simulink model "least_square_p3_3ordem"  (Simulink 10.3)
settings: Solver=VariableStepAuto  StartTime=0.0  StopTime=10.0  RelTol=1e-3
values from neighbouring files (symbols this model uses):
  Aq = 2    [sim_grad_norm_3ordem.m]
  As = 2    [sim_grad_norm.m]    (also in sim_grad_norm_3ordem.m = 0)
  DC = 1    [sim_grad_norm.m]    (also in sim_grad_norm_3ordem.m)
  kappa = 1e-9    (= 1e-09)    [sim_grad_norm.m]    (also in sim_grad_norm_3ordem.m = 1)
  lambda0 = 1    [sim_grad_norm.m]    (also in sim_grad_norm_3ordem.m)
  lambda1 = 2    [sim_grad_norm.m]    (also in sim_grad_norm_3ordem.m)
  lambda2 = 3    [sim_grad_norm.m]    (also in sim_grad_norm_3ordem.m)
  P0 = eye(6)    [sim_grad_norm.m]    (also in sim_grad_norm_3ordem.m = 1*eye(6))
  st = 0.01    [sim_grad_norm.m]    (also in sim_grad_norm_3ordem.m)
  theta0 = [0;0;0;0;0;0]    [sim_grad_norm.m]    (also in sim_grad_norm_3ordem.m)
  theta_star2 = [b0; b1; b2; a0; a1;a2]    [sim_grad_norm.m]    (also in sim_grad_norm_3ordem.m)
  wq = 0.1*pi    (= 0.314159265359)    [sim_grad_norm_3ordem.m]
  ws = 0.1*pi    (= 0.314159265359)    [sim_grad_norm.m]    (also in sim_grad_norm_3ordem.m = 3.14159265359)
libraries: cstblocks x1
settings Model: LogicAnalyzerSignalOrdering=70bf5b3e-6542-4105-83ca-980c629f65ae,9c30bcda-f0a5-4d45-8ce2-3a7fb53d1df5,0cef303f-29ae-401b-9088-eb7ee3a5d8ba,671b97e1-b0f3-4841-85b5-247d62c7300d,1faa530f-46b2-4af3-a98d-9f9eb6d754f3,8e948dc3-23ac-4809-bbbe-ffc7fe3ac31c,78968b27-08ba-45c6-8b8c-f5c28d25609d,488bf256-05e0-48c6-b81f-63abf945d574,54e25a1b-7dc9-472a-bcd8-055bce62d9cd,55c07523-ef82-4b70-b601-8332f774a6d4,291e4613-507b-452d-a549-2515bbd6c047,ac738118-fc15-4075-a2e0-d6a46a18733c  Creator=caioc  LastModifiedBy=caioc
settings SolverCC: AlgebraicLoopSolver=Auto
settings DataIOCC: SaveFormat=Dataset  SignalLoggingSaveFormat=Dataset  ReturnWorkspaceOutputs=on
settings OptimizationCC: ExpressionDepthLimit=128  LifeSpan=auto
settings DebuggingCC: UnderspecifiedInitializationDetection=Simplified  MergeDetectMultiDrivingBlocksExec=error  FcnCallInpInsideContextMsg=error  StateNameClashWarn=none  SFUnexpectedBacktrackingDiag=error  SFNoUnconditionalDefaultTransitionDiag=error  SFExecutionAtInitializationDiag=warning  SFMachineParentedDataDiag=error  ArithmeticOperatorsInVariantConditions=error
settings HardwareCC: ProdBitPerPointer=64  ProdBitPerSizeT=64  ProdBitPerPtrDiffT=64  ProdLargestAtomicFloat=Float  ProdIntDivRoundTo=Zero  ProdEndianess=LittleEndian  ProdWordSize=64  ProdHWDeviceType=Intel->x86-64 (Windows64)
settings ModelReferenceCC: PropagateSignalLabelsOutOfModel=on
settings SFSimCC: SimUseLocalCustomCode=on  CustomCodeUndefinedFunction=FilterOut
settings RTWCC: RTWUseLocalCustomCode=on
settings CodeAppCC: StateflowObjectComments=off
settings GRTTargetCC: TargetLangStandard=C99 (ISO)  CombineOutputUpdateFcns=on  GRTInterface=off
settings ConfigComp: CovMetricSettings=dwe  CovSaveCumulativeToWorkspaceVar=off  CovSaveSingleToWorkspaceVar=off  CovExternalEMLEnable=on

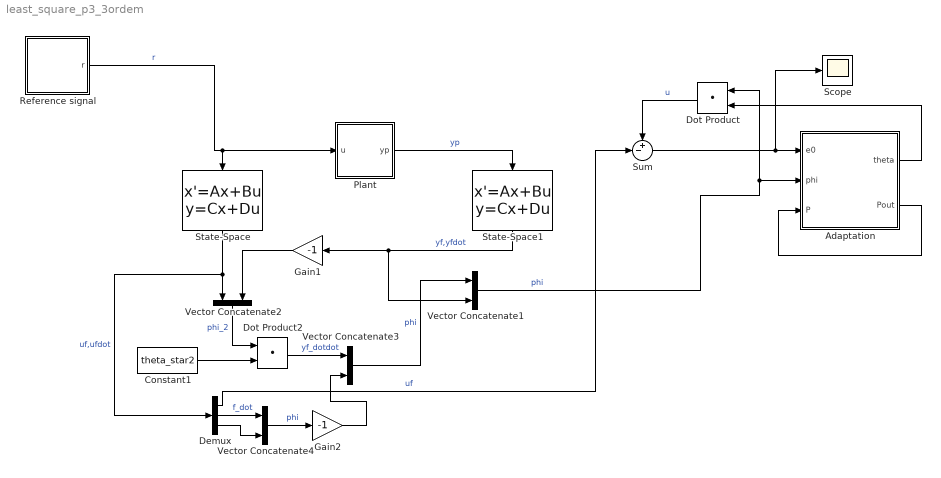
== system least_square_p3_3ordem ==
  Adaptation : Subsystem
  Constant1 : Constant  Value=theta_star2
  Demux : Demux  Outputs=3
  Dot Product : DotProduct  InputSameDT=on  OutDataTypeStr=Inherit: Inherit via internal rule
  Dot Product2 : DotProduct  InputSameDT=on  OutDataTypeStr=Inherit: Inherit via internal rule
  Gain1 : Gain  Gain=-1
  Gain2 : Gain  Gain=-1
  Plant : Subsystem
  Reference signal : Subsystem
  Scope : Scope
  State-Space : StateSpace  A=[0 1 0;0 0 1; -lambda0 -lambda1 -lambda2]  B=[0; 0; 1]  C=[1 0 0;0 1 0; 0 0 1]  D=[0;0;0]  InitialCondition=0
  State-Space1 : StateSpace  A=[0 1 0;0 0 1; -lambda0 -lambda1 -lambda2]  B=[0; 0; 1]  C=[1 0 0;0 1 0; 0 0 1]  D=[0;0;0]  InitialCondition=0
  Sum : Sum  Inputs=+-|
  Vector Concatenate{1..4} (4 alike) : Concatenate
  wires:
  Reference signal/1(r) -> State-Space/1, Plant/1(u)  "r"
  Sum/1 -> Scope/1, Adaptation/1(e0)
  Adaptation/1(theta) -> Dot Product/2
  Dot Product/1 -> Sum/1  "u"
  Plant/1(yp) -> State-Space1/1  "yp"
  Adaptation/2(Pout) -> Adaptation/3(P)
  Demux/1 -> Sum/2  "uf"
  Vector Concatenate2/1 -> Dot Product2/1  "phi_2"
  Gain1/1 -> Vector Concatenate2/2
  Dot Product2/1 -> Vector Concatenate3/1  "yf_dotdot"
  Constant1/1 -> Dot Product2/2
  Vector Concatenate3/1 -> Vector Concatenate1/1  "phi"
  State-Space/1 -> Vector Concatenate2/1, Demux/1  "uf,ufdot"
  Vector Concatenate1/1 -> Adaptation/2(phi), Dot Product/1  "phi"
  State-Space1/1 -> Vector Concatenate1/2, Gain1/1  "yf,yfdot"
  Gain2/1 -> Vector Concatenate3/2
  Vector Concatenate4/1 -> Gain2/1  "phi"
  Demux/3 -> Vector Concatenate4/2
  Demux/2 -> Vector Concatenate4/1  "f_dot"

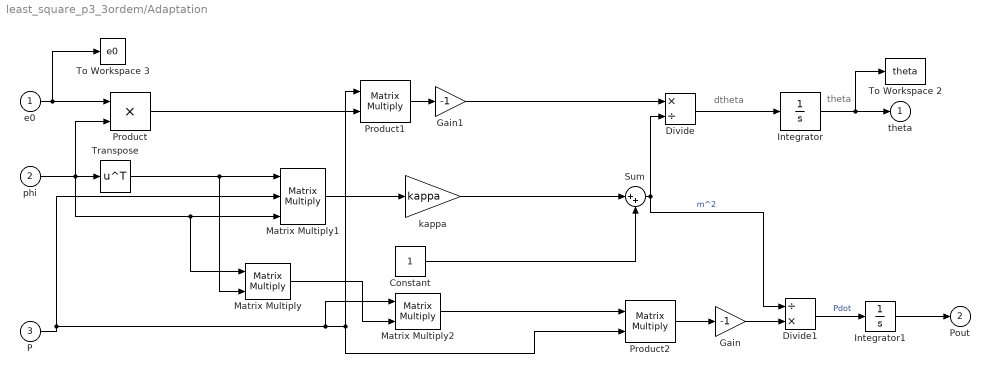
== system least_square_p3_3ordem/Adaptation ==
  note: theta
  note: dtheta
  e0 : Inport  PortDimensions=1
  phi : Inport  Port=2
  P : Inport  Port=3
  Constant : Constant
  Divide : Product  Inputs=*/
  Divide1 : Product  Inputs=/*
  Gain : Gain  Gain=-1
  Gain1 : Gain  Gain=-1
  Integrator : Integrator  InitialCondition=theta0
  Integrator1 : Integrator  InitialCondition=P0
  Matrix Multiply : Product  Multiplication=Matrix(*)
  Matrix Multiply1 : Product  Inputs=3  Multiplication=Matrix(*)
  Matrix Multiply2 : Product  Multiplication=Matrix(*)
  Product : Product  InputSameDT=on  RndMeth=Zero  SaturateOnIntegerOverflow=on  OutDataTypeStr=Inherit: Same as first input
  Product1 : Product  Multiplication=Matrix(*)
  Product2 : Product  Multiplication=Matrix(*)
  Sum : Sum  Inputs=|++
  To Workspace 2 : ToWorkspace  VariableName=theta  SampleTime=st
  To Workspace 3 : ToWorkspace  VariableName=e0  SampleTime=st
  Transpose : Math  Operator=transpose  SaturateOnIntegerOverflow=on
  kappa : Gain  Gain=kappa  SaturateOnIntegerOverflow=on  OutDataTypeStr=Inherit: Same as input  ParamDataTypeStr=Inherit: Same as input
  theta : Outport  InitialOutput=0  VectorParamsAs1DForOutWhenUnconnected=off
  Pout : Outport  Port=2  InitialOutput=0  VectorParamsAs1DForOutWhenUnconnected=off
  wires:
  Integrator/1 -> To Workspace 2/1, theta/1
  Divide/1 -> Integrator/1
  e0/1 -> Product/1, To Workspace 3/1
  Product1/1 -> Gain1/1
  Product/1 -> Product1/2
  phi/1 -> Matrix Multiply/1, Matrix Multiply1/3, Transpose/1, Product/2
  Constant/1 -> Sum/2
  kappa/1 -> Sum/1
  Sum/1 -> Divide1/1, Divide/2  "m^2"
  P/1 -> Matrix Multiply2/1, Product2/2, Product1/1, Matrix Multiply1/2
  Product2/1 -> Gain/1
  Matrix Multiply/1 -> Matrix Multiply2/2
  Transpose/1 -> Matrix Multiply1/1, Matrix Multiply/2
  Matrix Multiply1/1 -> kappa/1
  Integrator1/1 -> Pout/1
  Gain1/1 -> Divide/1
  Matrix Multiply2/1 -> Product2/1
  Gain/1 -> Divide1/2
  Divide1/1 -> Integrator1/1  "Pdot"

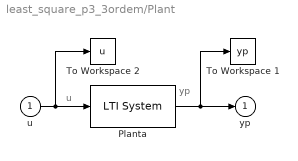
== system least_square_p3_3ordem/Plant ==
  note: yp
  note: u
  u : Inport
  Planta : cstblocks/LTI System  sys=P  IC=x0
  To Workspace 1 : ToWorkspace  VariableName=yp  SampleTime=st
  To Workspace 2 : ToWorkspace  VariableName=u  SampleTime=st
  yp : Outport  InitialOutput=0  VectorParamsAs1DForOutWhenUnconnected=off
  wires:
  u/1 -> To Workspace 2/1, Planta/1
  Planta/1 -> yp/1, To Workspace 1/1

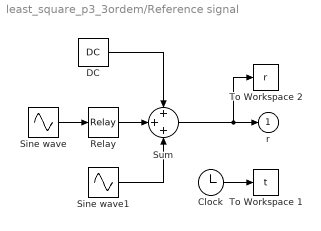
== system least_square_p3_3ordem/Reference signal ==
  Clock : Clock
  DC : Constant  Value=DC
  Relay : Relay  OnOutputValue=Aq  OffOutputValue=-Aq
  Sine wave : Sin  Frequency=wq  SampleTime=0
  Sine wave1 : Sin  Amplitude=As  Frequency=ws  SampleTime=0
  Sum : Sum  Inputs=+++  InputSameDT=on  SaturateOnIntegerOverflow=on  OutDataTypeStr=Inherit: Same as first input
  To Workspace 1 : ToWorkspace  VariableName=t  SampleTime=st
  To Workspace 2 : ToWorkspace  VariableName=r  SampleTime=st
  r : Outport  InitialOutput=0  VectorParamsAs1DForOutWhenUnconnected=off
  wires:
  Clock/1 -> To Workspace 1/1
  Sine wave1/1 -> Sum/3
  Sine wave/1 -> Relay/1
  Relay/1 -> Sum/2
  DC/1 -> Sum/1
  Sum/1 -> r/1, To Workspace 2/1
